simulink model "Galvo_compare_cc_and_nocc_v1"  (R2013a)
settings: Solver=ode45  StartTime=0.0  StopTime=5e-3  FixedStep=FS  MaxStep=1e-4  RelTol=1e-3  AbsTol=1e-5
PreLoadFcn:
  | vname=@(x) inputname(1);
  | paramCtrl=evalin('base','paramCtrl;');
  | I_LIM=str2num(paramCtrl.I_LIM);
  | Kbc=str2num(paramCtrl.Kbc);
  | FS=evalin('base','FS;');
InitFcn:
  | I_LIM=str2num(paramCtrl.I_LIM);
  | Kbc=str2num(paramCtrl.Kbc);
  | %FS=evalin('base','FS;');
  | 
  | %%%%%%  set scope time range
  | T_STOP=str2num(get_param(gcs,'StopTime'));
  | if numel(T_STOP) > 1
  |    T_STOP=T_STOP(2);
  | else
  |    T_STOP=T_STOP(1);
  | end
  | T_STOP=num2str(T_STOP);
  | 
  | %%%%%%  set scope time range in system @init_callback_fct
  | T_STOP=num2str(str2num(get_param(gcs,'StopTime')));
  | 
  | childs = allchild(0);
  | sol=strfind(upper(get(allchild(0),'Tag')),'VIEWER_PARAMETERS');
  | 
  | if iscell(sol)
  |    ind=find(~cellfun(@isempty, strfind(upper(get(allchild(0),'Tag')),'VIEWER_PARAMETERS')));
  | else
  |    ind=sol;
  | end
  | %ind=find(~cellfun(@isempty, {strfind(upper(get(allchild(0),'Tag')),'VIEWER_PARAMETERS'),[]}))
  | if ~isempty(ind)
  |     set_param(getfield(get(childs(ind),'UserData'),'block'),'TimeRange',T_STOP);
  |     get_param(getfield(get(childs(ind),'UserData'),'block'),'TimeRange');
  | else
  |     warning(sprintf('VIEWER_PARAMETERS object not found\nOpen the config dialog by hand for the first sim start'))
  | end
StartFcn:
  | I_LIM=str2num(paramCtrl.I_LIM);
  | Kbc=str2num(paramCtrl.Kbc);
  | %FS=evalin('base','FS;');
undefined symbols (not defined in the file or in its folder): JR, KBM, KFR, KMT, KTB, Lc, Rc, Rsh
libraries: simulink x5, dspsigops x1
settings Model: BufferReuse=off  Creator=mainster  LastModifiedBy=mainster
settings SolverCC: AutoInsertRateTranBlk=on
settings DataIOCC: LimitDataPoints=off  SaveOutput=off  SaveTime=off
settings OptimizationCC: BlockReduction=off  OptimizeBlockIOStorage=off  BufferReuse=off  ExpressionFolding=off  LocalBlockOutputs=off
settings ModelReferenceCC: ModelReferenceNumInstancesAllowed=Single

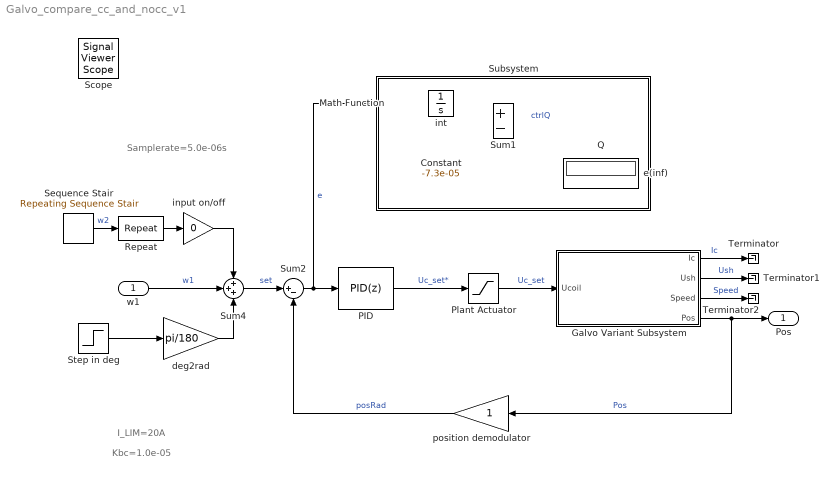
== system Galvo_compare_cc_and_nocc_v1 ==
  note: I_LIM=20A
  note: Kbc=1.0e-05
  note: Samplerate=5.0e-06s
  w1 : Inport  SampleTime=FS
  Constant : Constant  Value=-7.3e-05  SampleTime=FS
  Galvo Variant Subsystem : Subsystem  Variant=on  OverrideUsingVariant=NoCC
  Math Function : Math  Operator=square  OutputSignalType=real  SampleTime=FS  SaturateOnIntegerOverflow=on
  PID : simulink/Continuous/PID Controller  Controller=PID  TimeDomain=Discrete-time  SampleTime=FS  IntegratorMethod=Forward Euler  FilterMethod=Forward Euler  Form=Ideal  P=24.8595069348583  I=18.0024129719126  D=0.000624760000899868  N=11350.149813225  InitialConditionSource=internal  InitialConditionForIntegrator=0  InitialConditionForFilter=0  ExternalReset=none  IgnoreLimit=on  LimitOutput=on  UpperSaturationLimit=30  LowerSaturationLimit=-30  LinearizeAsGain=off  AntiWindupMode=back-calculation  Kb=0.1  TrackingMode=off  Kt=0  PParamMin=[]  PParamMax=[]  IParamMin=[]  IParamMax=[]  DParamMin=[]  DParamMax=[]  NParamMin=[]  NParamMax=[]  KbParamMin=[]  KbParamMax=[]  KtParamMin=[]  KtParamMax=[]  POutMin=[]  POutMax=[]  IOutMin=[]  IOutMax=[]  DOutMin=[]  DOutMax=[]  NOutMin=[]  NOutMax=[]  KbOutMin=[]  KbOutMax=[]  KtOutMin=[]  KtOutMax=[]  IntegratorOutMin=[]  IntegratorOutMax=[]  FilterOutMin=[]  FilterOutMax=[]  SumOutMin=[]  SumOutMax=[]  SumI1OutMin=[]  SumI1OutMax=[]  SumI2OutMin=[]  SumI2OutMax=[]  SumI3OutMin=[]  SumI3OutMax=[]  SumDOutMin=[]  SumDOutMax=[]  SaturationOutMin=[]  SaturationOutMax=[]  IntegratorContinuousStateAttributes=''  IntegratorStateMustResolveToSignalObject=off  IntegratorRTWStateStorageClass=Auto  FilterContinuousStateAttributes=''  FilterStateMustResolveToSignalObject=off  FilterRTWStateStorageClass=Auto
      settings: AttributesFormatString=AWM=%<AntiWindupMode>\nD=%<D>\nI=%<I>\nN=%<N>\nP=%<P>\nLimit=+-%<UpperSaturationLimit>
  Plant Actuator : Saturate  UpperLimit=30  LowerLimit=-30  SampleTime=FS
  Q : Display
      settings: Format=short_e
  Repeat : dspsigops/Repeat  N=length(str2num(get_param([gcs '/Sequence Stair'], 'OutValues')))  InputProcessing=Columns as channels (frame based)  RateOptions=Allow multirate processing  ic=0  mode=Unused parameter value
  Sequence Stair : simulink/Sources/Repeating Sequence Stair  OutValues="pi/180*[-10     0    14     3    12     9     3    -9     6 1 2   -15     5     6     8    14    17].'"  tsamp=(str2num(get_param(gcs,'StopTime')) / length(str2num(get_param([gcs '/Sequence Stair'], 'OutValues'))))  OutMin=[]  OutMax=[]  OutDataTypeStr=double  OutputDataTypeScalingMode=double  OutDataType=fixdt(0,8)  ConRadixGroup=Best Precision: Vector-wise  OutScaling=2^-12
  Step in deg : Step  Time=1e-3  After=10  SampleTime=FS  ZeroCross=off
      settings: AttributesFormatString=Ampl.: %<After>\ntime:%<Time>
  Subsystem : Subsystem
      mask Display: text(.05,.05,['{\fontsize{14}\it\bfL_2 Quality}'],'horizontalAlignment','left','verticalAlignment','bottom','texmode','on')
  Sum1 : Sum  Inputs=+-  SampleTime=FS
  Sum2 : Sum  Inputs=|+-  SampleTime=FS
  Sum4 : Sum  Inputs=+++  SampleTime=FS
  Terminator : Terminator
  Terminator1 : Terminator
  Terminator2 : Terminator
  deg2rad : Gain  Gain=pi/180  SampleTime=FS
  e(inf) : Display
      settings: Format=short_e
  input on/off : Gain  Gain=0  SampleTime=FS
  int : Integrator
  position demodulator : Gain  SampleTime=FS
  Pos : Outport  SampleTime=FS
  Scope : SignalViewerScope  IOType=viewer  NumInputPorts=4  LegendLocations=|  RefreshTime=0.033391
      | 0.80191     0.91082     0.13206    0.042716
      | 0.82377     0.69454      0.1102    0.023981
      |  0.7582      0.4408     0.17577    0.042716
      | 0.81284     0.22572     0.12113    0.023981
      settings: ShowLegends=on  TimeRange=0.005  YMin=0~-0.05~-5~-4  YMax=0.2~0.2~30~10
  wires:
  w1/1 -> Sum4/2  "w1"
  PID/1 -> Plant Actuator/1  "Uc_set*"
  Plant Actuator/1 -> Galvo Variant Subsystem/1(Ucoil)  "Uc_set"
  Sequence Stair/1 -> Repeat/1  "w2"
  Repeat/1 -> input on/off/1
  position demodulator/1 -> Sum2/2  "posRad"
  Sum2/1 -> Math Function/1, PID/1  "e"
  Sum4/1 -> Sum2/1  "set"
  Step in deg/1 -> deg2rad/1
  input on/off/1 -> Sum4/1
  deg2rad/1 -> Sum4/3
  int/1 -> Sum1/1
  Math Function/1 -> int/1
  Sum1/1 -> Q/1  "ctrlQ"
  Constant/1 -> e(inf)/1, Sum1/2
  Galvo Variant Subsystem/4(Pos) -> position demodulator/1, Pos/1  "Pos"
  Galvo Variant Subsystem/3(Speed) -> Terminator2/1  "Speed"
  Galvo Variant Subsystem/2(Ush) -> Terminator1/1  "Ush"
  Galvo Variant Subsystem/1(Ic) -> Terminator/1  "Ic"

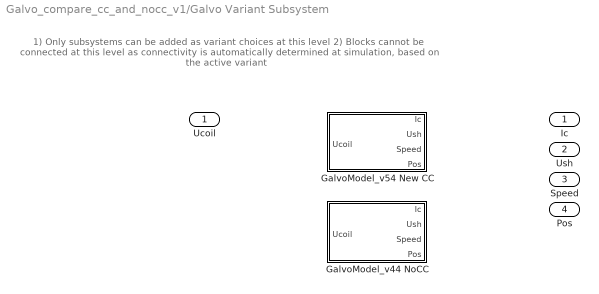
== system Galvo_compare_cc_and_nocc_v1/Galvo Variant Subsystem ==
  note: 1) Only subsystems can be added as variant choices at this level
      | 2) Blocks cannot be connected at this level as connectivity is
      | automatically determined at simulation, based on the active variant
  Ucoil : Inport
  GalvoModel_v44 NoCC : Subsystem  VariantControl=NoCC
  GalvoModel_v54 New CC : Subsystem  VariantControl=NewCC
  Ic : Outport
  Ush : Outport  Port=2
  Speed : Outport  Port=3
  Pos : Outport  Port=4

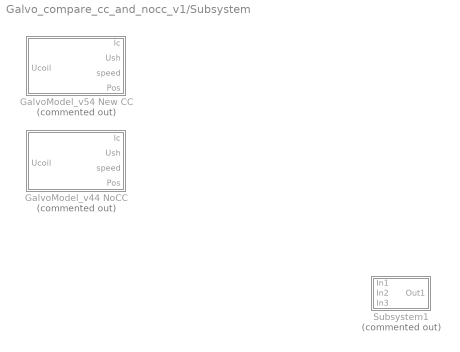
== system Galvo_compare_cc_and_nocc_v1/Subsystem ==
  GalvoModel_v44 NoCC : Subsystem  Commented=on  VariantControl=Variant1
  GalvoModel_v54 New CC : Subsystem  Commented=on  VariantControl=Variant
  Subsystem1 : Subsystem  Commented=on

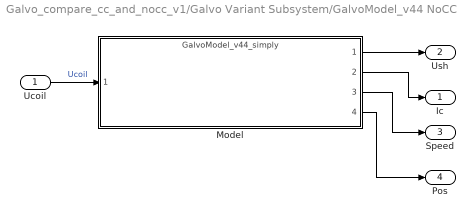
== system Galvo_compare_cc_and_nocc_v1/Galvo Variant Subsystem/GalvoModel_v44 NoCC ==
  Ucoil : Inport
  Model : ModelReference  ModelNameDialog=GalvoModel_v44_simply.slx  SimulationMode=Normal  ModelReferenceVersion=1.79  CopyOfModelName=GalvoModel_v44_simply.slx  DefaultDataLogging=on
  Ic : Outport
  Ush : Outport  Port=2
  Speed : Outport  Port=3
  Pos : Outport  Port=4
  wires:
  Ucoil/1 -> Model/1  "Ucoil"
  Model/1 -> Ush/1
  Model/2 -> Ic/1
  Model/3 -> Speed/1
  Model/4 -> Pos/1

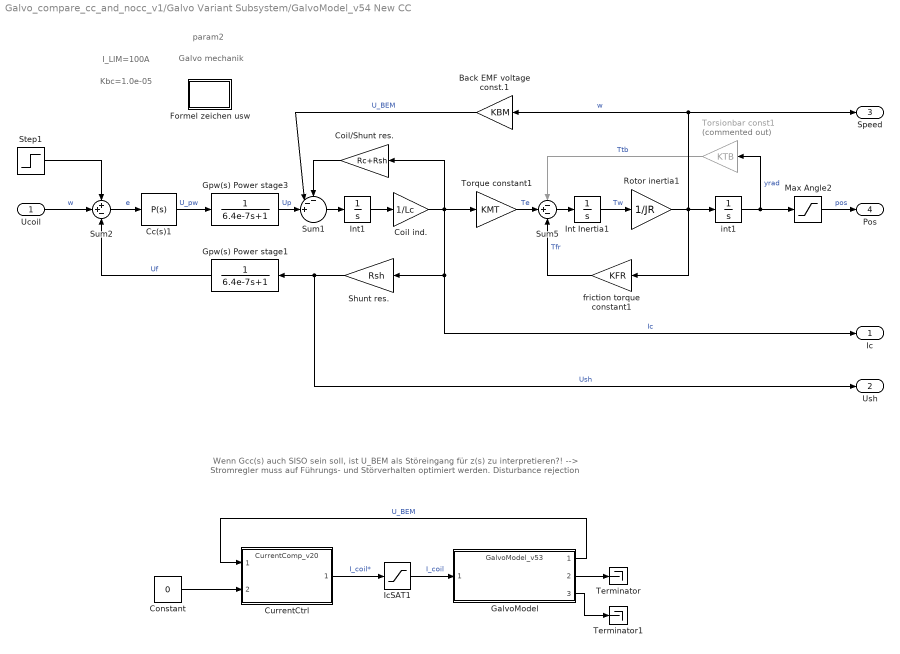
== system Galvo_compare_cc_and_nocc_v1/Galvo Variant Subsystem/GalvoModel_v54 New CC ==
  note: Wenn Gcc(s) auch SISO sein soll, ist U_BEM als Störeingang für z(s) zu interpretieren?!
      | --> Stromregler muss auf Führungs- und Störverhalten optimiert werden.
      | Disturbance rejection
  note: param2
  note: Galvo mechanik
  note: I_LIM=100A
  note: Kbc=1.0e-05
  Ucoil : Inport
  Back EMF voltage const.1 : Gain  Gain=KBM
  Cc(s)1 : simulink/Continuous/PID Controller  Controller=P  TimeDomain=Continuous-time  SampleTime=1  IntegratorMethod=Forward Euler  FilterMethod=Forward Euler  Form=Ideal  P=1.04148381747473  I=14540.01765706  D=0  N=100  InitialConditionSource=internal  InitialConditionForIntegrator=0  InitialConditionForFilter=0  ExternalReset=none  LimitOutput=off  UpperSaturationLimit=inf  LowerSaturationLimit=-inf  LinearizeAsGain=on  AntiWindupMode=none  Kb=1  TrackingMode=off  Kt=1  PParamMin=[]  PParamMax=[]  IParamMin=[]  IParamMax=[]  DParamMin=[]  DParamMax=[]  NParamMin=[]  NParamMax=[]  KbParamMin=[]  KbParamMax=[]  KtParamMin=[]  KtParamMax=[]  POutMin=[]  POutMax=[]  IOutMin=[]  IOutMax=[]  DOutMin=[]  DOutMax=[]  NOutMin=[]  NOutMax=[]  KbOutMin=[]  KbOutMax=[]  KtOutMin=[]  KtOutMax=[]  IntegratorOutMin=[]  IntegratorOutMax=[]  FilterOutMin=[]  FilterOutMax=[]  SumOutMin=[]  SumOutMax=[]  SumI1OutMin=[]  SumI1OutMax=[]  SumI2OutMin=[]  SumI2OutMax=[]  SumI3OutMin=[]  SumI3OutMax=[]  SumDOutMin=[]  SumDOutMax=[]  SaturationOutMin=[]  SaturationOutMax=[]  IntegratorContinuousStateAttributes=''  IntegratorStateMustResolveToSignalObject=off  IntegratorRTWStateStorageClass=Auto  FilterContinuousStateAttributes=''  FilterStateMustResolveToSignalObject=off  FilterRTWStateStorageClass=Auto
  Coil ind. : Gain  Gain=1/Lc
  Coil/Shunt res. : Gain  Gain=Rc+Rsh
  Constant : Constant  Value=0
  CurrentCtrl : ModelReference  ModelNameDialog=CurrentComp_v20.slx  SimulationMode=Normal  Variant=on  OverrideUsingVariant=cc_v20  ModelReferenceVersion=1.99  CopyOfModelName=CurrentComp_v20.slx  DefaultDataLogging=on
      mask Display:
      | str=sprintf('%s',get(gcbh,'ModelName'));
      | port_label('input', 2, 'I_{Set Coil}','texmode','on')
      | color('red');
      | port_label('input', 1, 'U_{BEM}','texmode','on')
      | color('black');
      | port_label('output', 1, 'I_{Coil}','texmode','on')
      | %text(.05,.98,['{\fontsize{12}\it\bf' strrep(str,'_',' ') '}'],'horizontalAlignment','left','verticalAlignment','top','texmode','on')
      | text(.95,0.95,['{\fontsize{12}\it\bfG_{cc}(s)}'],'horizontalAlignment','right','verticalAlignment','top','texmode','on')
      | %text(.15,.05,['{\fontsize{10}\itmechanics}'],'horizontalAlignment','left','verticalAlignment','bottom','texmode','on')
  Formel zeichen usw : Subsystem
  GalvoModel : ModelReference  ModelNameDialog=GalvoModel_v53.slx  SimulationMode=Normal  Variant=on  OverrideUsingVariant=v53_neuer_cc  ModelReferenceVersion=1.62  CopyOfModelName=GalvoModel_v53.slx  DefaultDataLogging=on
      mask Display:
      | str=sprintf('%s',get(gcbh,'ModelName'));
      | port_label('input', 1, 'I_{Coil}','texmode','on')
      | color('blue');
      | port_label('output', 3, 'Pos','texmode','on')
      | color('black');
      | port_label('output', 2, 'Speed','texmode','on')
      | port_label('output', 1, 'U_{BEM}','texmode','on')
      | %text(.05,.98,['{\fontsize{12}\it\bf' strrep(str,'_',' ') '}'],'horizontalAlignment','left','verticalAlignment','top','texmode','on')
      | text(.015,.98,['{\fontsize{12}\it\bf' strrep(str,'_','\_') '}'],'horizontalAlignment','left','verticalAlignment','top','texmode','on')
      | text(.15,.05,['{\fontsize{10}\itmechanics}'],'horizontalAlignment','left','verticalAlignment','bottom','texmode','on')
  Gpw(s) Power stage1 : TransferFcn  Denominator=[6.4e-7 1]
  Gpw(s) Power stage3 : TransferFcn  Denominator=[6.4e-7 1]
  IcSAT1 : Saturate  UpperLimit=I_LIM  LowerLimit=-I_LIM
  Int Inertia1 : Integrator
  Int1 : Integrator
  Max Angle2 : Saturate  UpperLimit=20*pi/180  LowerLimit=-20*pi/180
      settings: AttributesFormatString=Max=%<UpperLimit>\nMin=%<LowerLimit>
  Rotor inertia1 : Gain  Gain=1/JR
  Shunt res. : Gain  Gain=Rsh
  Step1 : Step  Time=1e3  After=1*pi/180  SampleTime=0  ZeroCross=off
      settings: AttributesFormatString=Ampl.: %<After>
  Sum1 : Sum  Inputs=--+||
  Sum2 : Sum  Inputs=++-
  Sum5 : Sum  Inputs=-+-
  Terminator : Terminator
  Terminator1 : Terminator
  Torque constant1 : Gain  Gain=KMT
  Torsionbar const1 : Gain  Commented=on  Gain=KTB
  friction torque constant1 : Gain  Gain=KFR
  int1 : Integrator
  Ic : Outport
  Ush : Outport  Port=2
  Speed : Outport  Port=3
  Pos : Outport  Port=4
  wires:
  Step1/1 -> Sum2/1
  Max Angle2/1 -> Pos/1  "pos"
  Sum2/1 -> Cc(s)1/1  "e"
  Coil/Shunt res./1 -> Sum1/1
  Sum1/1 -> Int1/1
  Int1/1 -> Coil ind./1
  Cc(s)1/1 -> Gpw(s) Power stage3/1  "U_pw"
  Gpw(s) Power stage3/1 -> Sum1/3  "Up"
  int1/1 -> Max Angle2/1, Torsionbar const1/1  "yrad"
  Torque constant1/1 -> Sum5/2  "Te"
  Torsionbar const1/1 -> Sum5/1  "Ttb"
  Int Inertia1/1 -> Rotor inertia1/1  "Tw"
  Sum5/1 -> Int Inertia1/1
  Rotor inertia1/1 -> int1/1, Speed/1, Back EMF voltage const.1/1, friction torque constant1/1  "w"
  friction torque constant1/1 -> Sum5/3  "Tfr"
  Coil ind./1 -> Ic/1, Shunt res./1, Torque constant1/1, Coil/Shunt res./1  "Ic"
  Back EMF voltage const.1/1 -> Sum1/2  "U_BEM"
  Gpw(s) Power stage1/1 -> Sum2/3  "Uf"
  Ucoil/1 -> Sum2/2  "w"
  Shunt res./1 -> Ush/1, Gpw(s) Power stage1/1  "Ush"
  GalvoModel/1 -> CurrentCtrl/1  "U_BEM"
  CurrentCtrl/1 -> IcSAT1/1  "I_coil*"
  IcSAT1/1 -> GalvoModel/1  "I_coil"
  Constant/1 -> CurrentCtrl/2
  GalvoModel/2 -> Terminator/1
  GalvoModel/3 -> Terminator1/1

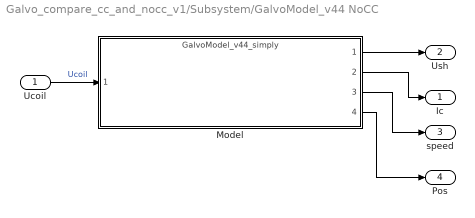
== system Galvo_compare_cc_and_nocc_v1/Subsystem/GalvoModel_v44 NoCC ==
  Ucoil : Inport
  Model : ModelReference  ModelNameDialog=GalvoModel_v44_simply.slx  SimulationMode=Normal  ModelReferenceVersion=1.79  CopyOfModelName=GalvoModel_v44_simply.slx  DefaultDataLogging=on
  Ic : Outport
  Ush : Outport  Port=2
  speed : Outport  Port=3
  Pos : Outport  Port=4
  wires:
  Ucoil/1 -> Model/1  "Ucoil"
  Model/1 -> Ush/1
  Model/2 -> Ic/1
  Model/3 -> speed/1
  Model/4 -> Pos/1

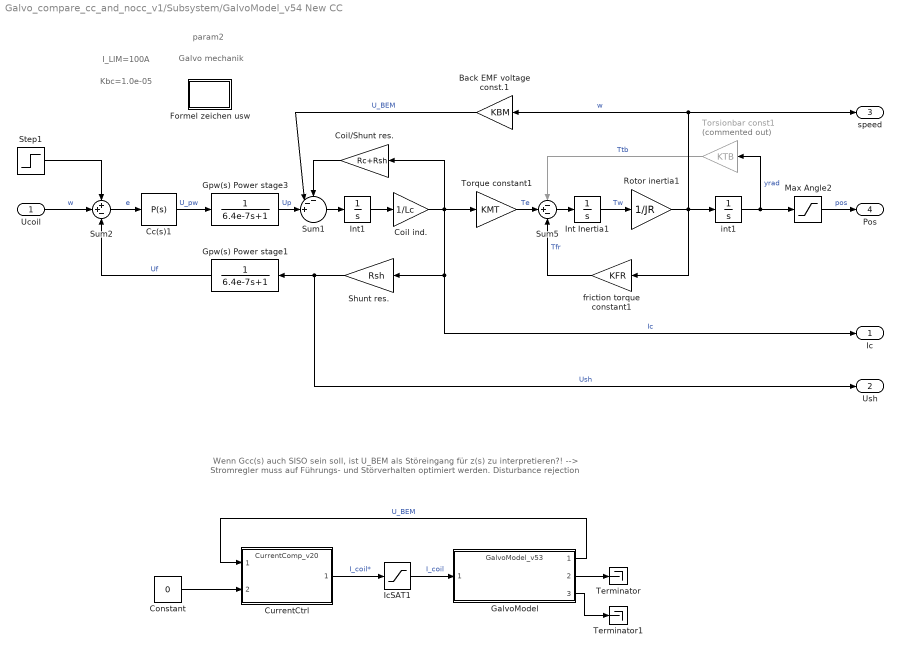
== system Galvo_compare_cc_and_nocc_v1/Subsystem/GalvoModel_v54 New CC ==
  note: Wenn Gcc(s) auch SISO sein soll, ist U_BEM als Störeingang für z(s) zu interpretieren?!
      | --> Stromregler muss auf Führungs- und Störverhalten optimiert werden.
      | Disturbance rejection
  note: param2
  note: Galvo mechanik
  note: I_LIM=100A
  note: Kbc=1.0e-05
  Ucoil : Inport
  Back EMF voltage const.1 : Gain  Gain=KBM
  Cc(s)1 : simulink/Continuous/PID Controller  Controller=P  TimeDomain=Continuous-time  SampleTime=1  IntegratorMethod=Forward Euler  FilterMethod=Forward Euler  Form=Ideal  P=5.91984122843419  I=14540.01765706  D=0  N=100  InitialConditionSource=internal  InitialConditionForIntegrator=0  InitialConditionForFilter=0  ExternalReset=none  LimitOutput=off  UpperSaturationLimit=inf  LowerSaturationLimit=-inf  LinearizeAsGain=on  AntiWindupMode=none  Kb=1  TrackingMode=off  Kt=1  PParamMin=[]  PParamMax=[]  IParamMin=[]  IParamMax=[]  DParamMin=[]  DParamMax=[]  NParamMin=[]  NParamMax=[]  KbParamMin=[]  KbParamMax=[]  KtParamMin=[]  KtParamMax=[]  POutMin=[]  POutMax=[]  IOutMin=[]  IOutMax=[]  DOutMin=[]  DOutMax=[]  NOutMin=[]  NOutMax=[]  KbOutMin=[]  KbOutMax=[]  KtOutMin=[]  KtOutMax=[]  IntegratorOutMin=[]  IntegratorOutMax=[]  FilterOutMin=[]  FilterOutMax=[]  SumOutMin=[]  SumOutMax=[]  SumI1OutMin=[]  SumI1OutMax=[]  SumI2OutMin=[]  SumI2OutMax=[]  SumI3OutMin=[]  SumI3OutMax=[]  SumDOutMin=[]  SumDOutMax=[]  SaturationOutMin=[]  SaturationOutMax=[]  IntegratorContinuousStateAttributes=''  IntegratorStateMustResolveToSignalObject=off  IntegratorRTWStateStorageClass=Auto  FilterContinuousStateAttributes=''  FilterStateMustResolveToSignalObject=off  FilterRTWStateStorageClass=Auto
  Coil ind. : Gain  Gain=1/Lc
  Coil/Shunt res. : Gain  Gain=Rc+Rsh
  Constant : Constant  Value=0
  CurrentCtrl : ModelReference  ModelNameDialog=CurrentComp_v20.slx  SimulationMode=Normal  Variant=on  OverrideUsingVariant=cc_v20  ModelReferenceVersion=1.99  CopyOfModelName=CurrentComp_v20.slx  DefaultDataLogging=on
      mask Display:
      | str=sprintf('%s',get(gcbh,'ModelName'));
      | port_label('input', 2, 'I_{Set Coil}','texmode','on')
      | color('red');
      | port_label('input', 1, 'U_{BEM}','texmode','on')
      | color('black');
      | port_label('output', 1, 'I_{Coil}','texmode','on')
      | %text(.05,.98,['{\fontsize{12}\it\bf' strrep(str,'_',' ') '}'],'horizontalAlignment','left','verticalAlignment','top','texmode','on')
      | text(.95,0.95,['{\fontsize{12}\it\bfG_{cc}(s)}'],'horizontalAlignment','right','verticalAlignment','top','texmode','on')
      | %text(.15,.05,['{\fontsize{10}\itmechanics}'],'horizontalAlignment','left','verticalAlignment','bottom','texmode','on')
  Formel zeichen usw : Subsystem
  GalvoModel : ModelReference  ModelNameDialog=GalvoModel_v53.slx  SimulationMode=Normal  Variant=on  OverrideUsingVariant=v53_neuer_cc  ModelReferenceVersion=1.62  CopyOfModelName=GalvoModel_v53.slx  DefaultDataLogging=on
      mask Display:
      | str=sprintf('%s',get(gcbh,'ModelName'));
      | port_label('input', 1, 'I_{Coil}','texmode','on')
      | color('blue');
      | port_label('output', 3, 'Pos','texmode','on')
      | color('black');
      | port_label('output', 2, 'Speed','texmode','on')
      | port_label('output', 1, 'U_{BEM}','texmode','on')
      | %text(.05,.98,['{\fontsize{12}\it\bf' strrep(str,'_',' ') '}'],'horizontalAlignment','left','verticalAlignment','top','texmode','on')
      | text(.015,.98,['{\fontsize{12}\it\bf' strrep(str,'_','\_') '}'],'horizontalAlignment','left','verticalAlignment','top','texmode','on')
      | text(.15,.05,['{\fontsize{10}\itmechanics}'],'horizontalAlignment','left','verticalAlignment','bottom','texmode','on')
  Gpw(s) Power stage1 : TransferFcn  Denominator=[6.4e-7 1]
  Gpw(s) Power stage3 : TransferFcn  Denominator=[6.4e-7 1]
  IcSAT1 : Saturate  UpperLimit=I_LIM  LowerLimit=-I_LIM
  Int Inertia1 : Integrator
  Int1 : Integrator
  Max Angle2 : Saturate  UpperLimit=20*pi/180  LowerLimit=-20*pi/180
      settings: AttributesFormatString=Max=%<UpperLimit>\nMin=%<LowerLimit>
  Rotor inertia1 : Gain  Gain=1/JR
  Shunt res. : Gain  Gain=Rsh
  Step1 : Step  Time=1e3  After=1*pi/180  SampleTime=0  ZeroCross=off
      settings: AttributesFormatString=Ampl.: %<After>
  Sum1 : Sum  Inputs=--+||
  Sum2 : Sum  Inputs=++-
  Sum5 : Sum  Inputs=-+-
  Terminator : Terminator
  Terminator1 : Terminator
  Torque constant1 : Gain  Gain=KMT
  Torsionbar const1 : Gain  Commented=on  Gain=KTB
  friction torque constant1 : Gain  Gain=KFR
  int1 : Integrator
  Ic : Outport
  Ush : Outport  Port=2
  speed : Outport  Port=3
  Pos : Outport  Port=4
  wires:
  Step1/1 -> Sum2/1
  Max Angle2/1 -> Pos/1  "pos"
  Sum2/1 -> Cc(s)1/1  "e"
  Coil/Shunt res./1 -> Sum1/1
  Sum1/1 -> Int1/1
  Int1/1 -> Coil ind./1
  Cc(s)1/1 -> Gpw(s) Power stage3/1  "U_pw"
  Gpw(s) Power stage3/1 -> Sum1/3  "Up"
  int1/1 -> Max Angle2/1, Torsionbar const1/1  "yrad"
  Torque constant1/1 -> Sum5/2  "Te"
  Torsionbar const1/1 -> Sum5/1  "Ttb"
  Int Inertia1/1 -> Rotor inertia1/1  "Tw"
  Sum5/1 -> Int Inertia1/1
  Rotor inertia1/1 -> int1/1, speed/1, Back EMF voltage const.1/1, friction torque constant1/1  "w"
  friction torque constant1/1 -> Sum5/3  "Tfr"
  Coil ind./1 -> Ic/1, Shunt res./1, Torque constant1/1, Coil/Shunt res./1  "Ic"
  Back EMF voltage const.1/1 -> Sum1/2  "U_BEM"
  Gpw(s) Power stage1/1 -> Sum2/3  "Uf"
  Ucoil/1 -> Sum2/2  "w"
  Shunt res./1 -> Ush/1, Gpw(s) Power stage1/1  "Ush"
  GalvoModel/1 -> CurrentCtrl/1  "U_BEM"
  CurrentCtrl/1 -> IcSAT1/1  "I_coil*"
  IcSAT1/1 -> GalvoModel/1  "I_coil"
  Constant/1 -> CurrentCtrl/2
  GalvoModel/2 -> Terminator/1
  GalvoModel/3 -> Terminator1/1

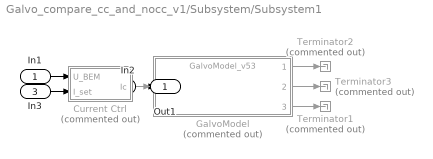
== system Galvo_compare_cc_and_nocc_v1/Subsystem/Subsystem1 ==
  In1 : Inport
  In2 : Inport  Port=2
  In3 : Inport  Port=3
  Current Ctrl : Subsystem  Commented=on
  GalvoModel : ModelReference  Commented=on  ModelNameDialog=GalvoModel_v53.slx  SimulationMode=Normal  OverrideUsingVariant=v53_neuer_cc  ModelReferenceVersion=1.62  CopyOfModelName=GalvoModel_v53.slx  DefaultDataLogging=on
      mask Display:
      | str=sprintf('%s',get(gcbh,'ModelName'));
      | port_label('input', 1, 'I_{Coil}','texmode','on')
      | color('blue');
      | port_label('output', 3, 'Pos','texmode','on')
      | color('black');
      | port_label('output', 2, 'Speed','texmode','on')
      | port_label('output', 1, 'U_{BEM}','texmode','on')
      | %text(.05,.98,['{\fontsize{12}\it\bf' strrep(str,'_',' ') '}'],'horizontalAlignment','left','verticalAlignment','top','texmode','on')
      | text(.015,.98,['{\fontsize{12}\it\bf' strrep(str,'_','\_') '}'],'horizontalAlignment','left','verticalAlignment','top','texmode','on')
      | text(.15,.05,['{\fontsize{10}\itmechanics}'],'horizontalAlignment','left','verticalAlignment','bottom','texmode','on')
  Terminator1 : Terminator  Commented=on
  Terminator2 : Terminator  Commented=on
  Terminator3 : Terminator  Commented=on
  Out1 : Outport
  wires:
  In2/1 -> GalvoModel/1
  In1/1 -> Current Ctrl/1(U_BEM)
  In3/1 -> Current Ctrl/2(I_set)
  Current Ctrl/1(Ic) -> Out1/1
  GalvoModel/3 -> Terminator1/1
  GalvoModel/2 -> Terminator3/1
  GalvoModel/1 -> Terminator2/1

== system Galvo_compare_cc_and_nocc_v1/Galvo Variant Subsystem/GalvoModel_v54 New CC/Formel zeichen usw ==
  note: Te: 		electrical torque, gen. by coils		[Nm]
      |  Ic: 			coil current							[A]
      |  Tfr:		rotor dynamic friction torque 		[Nm]
      |  Trb:		torsion bar torque					[Nm]
      |  Tw:		angular momentum				[Nm*s]
      |  w:			angular velocity 					[rad/s]
      |  yrad:		angular position 					[rad]
      |  ydeg:		angular position 					[°]
      |  Ucci:		current controller input				[V]
      |  Ucco:		current controller output			[V]
      |  Ush:		shunt voltage						[V]
  note: L_{c  }	coil inductance 							[H]
      |  R_{c  }	coil resistance							[\Omega]
      |  R_{SH }	current shunt resistance				[\Omega]
      |  J_{R  }	rotor inertia 							[kg*m²]
      |  K_{TB }	torsion bar torque const. 			[Nm/rad]
      |  K_{BM }	back EMF const.							[V*s/rad]
      |  K_{FR }	rotor dyn. friction torque const.	[Nm*s/rad]
      |  K_{MT }	el. magnetic torque const.			[Nm/A]
  note: balance of force: 	Te=Ttb+Tfr
      | 					Te - (Ttb+Tfr)=0  ->  no movement
      |
      |  integrate( 1 Nm )dt = 1 Nm*s
      |  (Nm*s)(kg*m²)⁻¹ = (N*s/kg)*m⁻¹ = m/(s*m) = rad

== system Galvo_compare_cc_and_nocc_v1/Subsystem/GalvoModel_v54 New CC/Formel zeichen usw ==
  note: Te: 		electrical torque, gen. by coils		[Nm]
      |  Ic: 			coil current							[A]
      |  Tfr:		rotor dynamic friction torque 		[Nm]
      |  Trb:		torsion bar torque					[Nm]
      |  Tw:		angular momentum				[Nm*s]
      |  w:			angular velocity 					[rad/s]
      |  yrad:		angular position 					[rad]
      |  ydeg:		angular position 					[°]
      |  Ucci:		current controller input				[V]
      |  Ucco:		current controller output			[V]
      |  Ush:		shunt voltage						[V]
  note: L_{c  }	coil inductance 							[H]
      |  R_{c  }	coil resistance							[\Omega]
      |  R_{SH }	current shunt resistance				[\Omega]
      |  J_{R  }	rotor inertia 							[kg*m²]
      |  K_{TB }	torsion bar torque const. 			[Nm/rad]
      |  K_{BM }	back EMF const.							[V*s/rad]
      |  K_{FR }	rotor dyn. friction torque const.	[Nm*s/rad]
      |  K_{MT }	el. magnetic torque const.			[Nm/A]
  note: balance of force: 	Te=Ttb+Tfr
      | 					Te - (Ttb+Tfr)=0  ->  no movement
      |
      |  integrate( 1 Nm )dt = 1 Nm*s
      |  (Nm*s)(kg*m²)⁻¹ = (N*s/kg)*m⁻¹ = m/(s*m) = rad

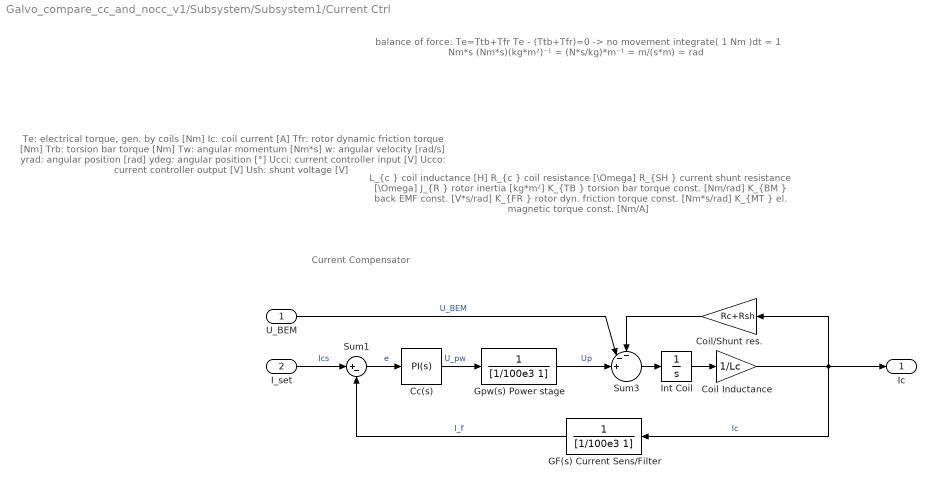
== system Galvo_compare_cc_and_nocc_v1/Subsystem/Subsystem1/Current Ctrl ==
  note: Current Compensator
  note: Te: 		electrical torque, gen. by coils		[Nm]
      |  Ic: 			coil current							[A]
      |  Tfr:		rotor dynamic friction torque 		[Nm]
      |  Trb:		torsion bar torque					[Nm]
      |  Tw:		angular momentum				[Nm*s]
      |  w:			angular velocity 					[rad/s]
      |  yrad:		angular position 					[rad]
      |  ydeg:		angular position 					[°]
      |  Ucci:		current controller input				[V]
      |  Ucco:		current controller output			[V]
      |  Ush:		shunt voltage						[V]
  note: L_{c  }	coil inductance 							[H]
      |  R_{c  }	coil resistance							[\Omega]
      |  R_{SH }	current shunt resistance				[\Omega]
      |  J_{R  }	rotor inertia 							[kg*m²]
      |  K_{TB }	torsion bar torque const. 			[Nm/rad]
      |  K_{BM }	back EMF const.							[V*s/rad]
      |  K_{FR }	rotor dyn. friction torque const.	[Nm*s/rad]
      |  K_{MT }	el. magnetic torque const.			[Nm/A]
  note: balance of force: 	Te=Ttb+Tfr
      | 					Te - (Ttb+Tfr)=0  ->  no movement
      |
      |  integrate( 1 Nm )dt = 1 Nm*s
      |  (Nm*s)(kg*m²)⁻¹ = (N*s/kg)*m⁻¹ = m/(s*m) = rad
  U_BEM : Inport
  I_set : Inport  Port=2
  Cc(s) : simulink/Continuous/PID Controller  Controller=PI  TimeDomain=Continuous-time  SampleTime=1  IntegratorMethod=Forward Euler  FilterMethod=Forward Euler  Form=Ideal  P=2.58986900309333  I=14540.01765706  D=0  N=100  InitialConditionSource=internal  InitialConditionForIntegrator=0  InitialConditionForFilter=0  ExternalReset=none  LimitOutput=off  UpperSaturationLimit=inf  LowerSaturationLimit=-inf  LinearizeAsGain=on  AntiWindupMode=none  Kb=1  TrackingMode=off  Kt=1  PParamMin=[]  PParamMax=[]  IParamMin=[]  IParamMax=[]  DParamMin=[]  DParamMax=[]  NParamMin=[]  NParamMax=[]  KbParamMin=[]  KbParamMax=[]  KtParamMin=[]  KtParamMax=[]  POutMin=[]  POutMax=[]  IOutMin=[]  IOutMax=[]  DOutMin=[]  DOutMax=[]  NOutMin=[]  NOutMax=[]  KbOutMin=[]  KbOutMax=[]  KtOutMin=[]  KtOutMax=[]  IntegratorOutMin=[]  IntegratorOutMax=[]  FilterOutMin=[]  FilterOutMax=[]  SumOutMin=[]  SumOutMax=[]  SumI1OutMin=[]  SumI1OutMax=[]  SumI2OutMin=[]  SumI2OutMax=[]  SumI3OutMin=[]  SumI3OutMax=[]  SumDOutMin=[]  SumDOutMax=[]  SaturationOutMin=[]  SaturationOutMax=[]  IntegratorContinuousStateAttributes=''  IntegratorStateMustResolveToSignalObject=off  IntegratorRTWStateStorageClass=Auto  FilterContinuousStateAttributes=''  FilterStateMustResolveToSignalObject=off  FilterRTWStateStorageClass=Auto
  Coil Inductance : Gain  Gain=1/Lc
  Coil/Shunt res. : Gain  Gain=Rc+Rsh
  GF(s) Current Sens/Filter : TransferFcn  Denominator=[1/100e3 1]
  Gpw(s) Power stage : TransferFcn  Denominator=[1/100e3 1]
  Int Coil : Integrator
  Sum1 : Sum  Inputs=|+-
  Sum3 : Sum  Inputs=--+||
  Ic : Outport
  wires:
  Cc(s)/1 -> Gpw(s) Power stage/1  "U_pw"
  GF(s) Current Sens/Filter/1 -> Sum1/2  "I_f"
  Coil/Shunt res./1 -> Sum3/1
  Sum3/1 -> Int Coil/1
  Gpw(s) Power stage/1 -> Sum3/3  "Up"
  Coil Inductance/1 -> Ic/1, GF(s) Current Sens/Filter/1, Coil/Shunt res./1  "Ic"
  I_set/1 -> Sum1/1  "Ics"
  Sum1/1 -> Cc(s)/1  "e"
  Int Coil/1 -> Coil Inductance/1
  U_BEM/1 -> Sum3/2  "U_BEM"
